simulink model "Simu_CA_CC_CC"  (R2024b)
settings: Solver=VariableStepAuto  StartTime=0.0  StopTime=10/60  RelTol=1e-3
libraries: spsDiodeLib x10, spsCurrentMeasurementLib x6, spsVoltageMeasurementLib x5, spsSeriesRLCBranchLib x2, spsACVoltageSourceLib x1, spsMeanLib x1, spsThreePhaseSourceLib x1, sps_lib x1
settings Model: Creator=usuario  LastModifiedBy=PC
settings OptimizationCC: ReuseModelBlockBuffer=off
settings RTWCC: GPUComputeCapability=3.5

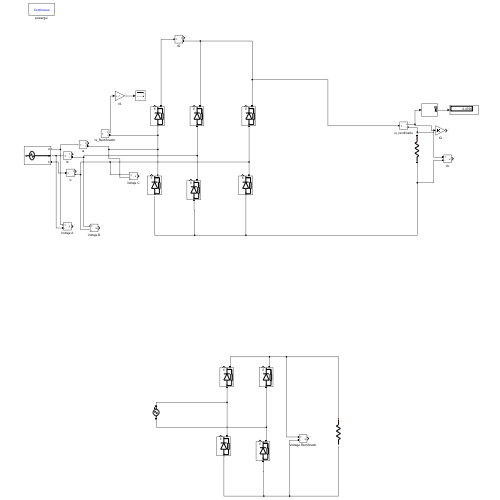
[thumbnail: Simulink's stored preview of the top-level diagram]
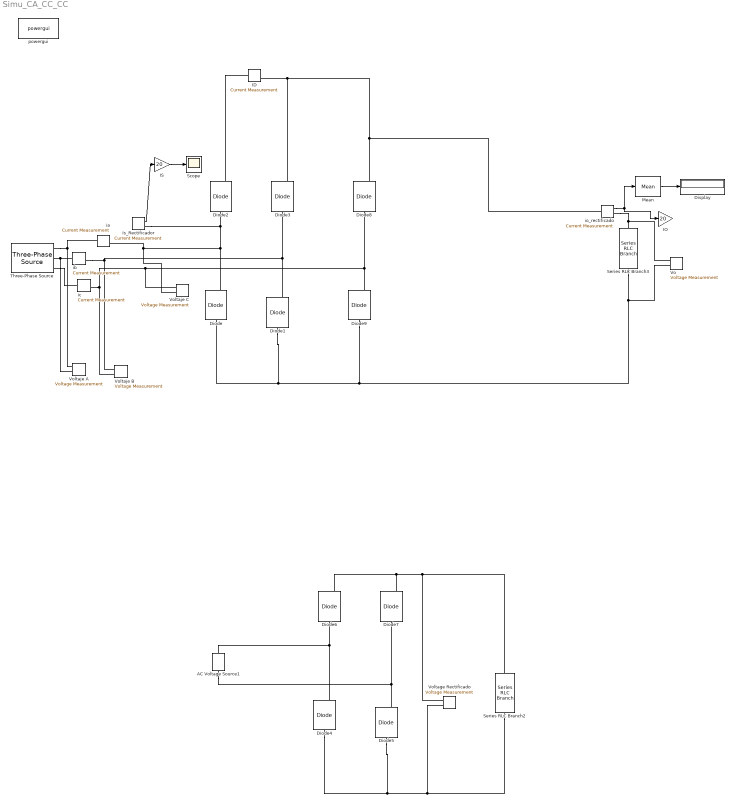
== system Simu_CA_CC_CC ==
  AC Voltage Source1 : spsACVoltageSourceLib/AC Voltage Source  Amplitude=105.56  Phase=0  Frequency=60  SampleTime=0  Measurements=None  BusType=swing  Pref=10e3  Qref=0  Qmin=-inf  Qmax=+inf
  Diode{,1..9} (10 alike) : spsDiodeLib/Diode  Ron=0.001  Lon=0  Vf=0.2  IC=0  UseSnubber=0  Rs=500  Cs=250e-9  Measurements=on
  Display : Display
  ID : spsCurrentMeasurementLib/Current Measurement  PhasorSimulation=off  OutputType=Complex  PSBequivalent=0
  IO : Gain  Gain=20
  IS : Gain  Gain=20
  Is_Rectificador : spsCurrentMeasurementLib/Current Measurement  PhasorSimulation=off  OutputType=Complex  PSBequivalent=0
  Mean : spsMeanLib/Mean  Freq=60  Vinit=0  Ts=0
  Scope : Scope
  Series RLC Branch2 : spsSeriesRLCBranchLib/Series RLC Branch  LConnTagsString=__new0  RConnTagsString=__new0  BranchType=R  Resistance=171  Inductance=1e-3  SetiL0=off  InitialCurrent=0  Capacitance=1e-6  Setx0=off  InitialVoltage=0  Measurements=Branch voltage and current
  Series RLC Branch3 : spsSeriesRLCBranchLib/Series RLC Branch  LConnTagsString=__new0  RConnTagsString=__new0  BranchType=R  Resistance=171  Inductance=1e-3  SetiL0=off  InitialCurrent=0  Capacitance=1e-6  Setx0=off  InitialVoltage=0  Measurements=Branch voltage and current
  Three-Phase Source : spsThreePhaseSourceLib/Three-Phase Source  InternalConnection=Yn  VoltagePhases=off  Voltage=60  PhaseAngle=0  Voltage_phases=[25e3 25e3 25e3]/sqrt(3)  PhaseAngles_phases=[0 -120 +120]  Frequency=60  NonIdealSource=on  SpecifyImpedance=off  Resistance=0  Inductance=0  ShortCircuitLevel=100e6  BaseVoltage=25e3  XRratio=7  BusType=swing  Pref=10e3  Qref=0  Prefabc=[10e3, 10e3, 10e3]  Qrefabc=[0, 0, 0]  Qmin=-inf  Qmax=inf
  Vo : spsVoltageMeasurementLib/Voltage Measurement  PhasorSimulation=off  OutputType=Complex  PSBequivalent=0
  Voltage Rectificado : spsVoltageMeasurementLib/Voltage Measurement  PhasorSimulation=off  OutputType=Complex  PSBequivalent=0
  Voltaje A : spsVoltageMeasurementLib/Voltage Measurement  PhasorSimulation=off  OutputType=Complex  PSBequivalent=0
  Voltaje B : spsVoltageMeasurementLib/Voltage Measurement  PhasorSimulation=off  OutputType=Complex  PSBequivalent=0
  Voltaje C : spsVoltageMeasurementLib/Voltage Measurement  PhasorSimulation=off  OutputType=Complex  PSBequivalent=0
  ia : spsCurrentMeasurementLib/Current Measurement  PhasorSimulation=off  OutputType=Complex  PSBequivalent=0
  ib : spsCurrentMeasurementLib/Current Measurement  PhasorSimulation=off  OutputType=Complex  PSBequivalent=0
  ic : spsCurrentMeasurementLib/Current Measurement  PhasorSimulation=off  OutputType=Complex  PSBequivalent=0
  io_rectificado : spsCurrentMeasurementLib/Current Measurement  PhasorSimulation=off  OutputType=Complex  PSBequivalent=0
  powergui : sps_lib/powergui  Priority=1  SimulationMode=Continuous  SampleTime=50e-6  frequency=60  Iterations=50  frequencyindice=60  Pbase=100e6  ErrMax=1e-4  UnitsV=kV  UnitsW=MW  buscounter=0  FunctionMessages=off  echomessages=off  EnableUseOfTLC=off  CurrentSourceSwitches=off  DisableSnubberDevices=off  DisableRonSwitches=off  DisableVfSwitches=off  DisplayEquations=off  AutomaticDiscreteSolvers=off  SolverType=Tustin/Backward Euler (TBE)  Interpol=off  ExternalGateDelay=off  methode=off  Ts=100  x0status=blocks  SPID=on  SwTol=0  HookPort=off  NonlinearTolerance=1e-4  nMaxIteration=100  ContinueOnMaxIteration=off  RestoreLinks=warning  ResistiveCurrentMeasurement=off  Frange=[0:2:500]  Ylog=off  Xlog=on  ShowGrid=off  save=off  variable=ZData  structure=0  ZoomFFT=off  StartTime=0.0  cycles=1  DisplayStyle=1  fundamental=60  FreqAxis=off  MaxFrequency=1000  frequencyindicesteady=1  RmsSteady=1  display=off
  wires:
  Mean/1 -> Display/1
  io_rectificado/1 -> IO/1, Mean/1
  Is_Rectificador/1 -> IS/1
  IS/1 -> Scope/1
  connections:
  Diode1/LConn1 -- Vo/LConn2 -- Series RLC Branch3/RConn1 -- Diode9/LConn1 -- Diode/LConn1
  Diode3/RConn1 -- io_rectificado/LConn1 -- Diode8/RConn1 -- ID/RConn1
  Diode/RConn1 -- ia/RConn1 -- Voltaje C/LConn2 -- Is_Rectificador/RConn1 -- Diode2/LConn1
  Diode1/RConn1 -- ib/RConn1 -- Voltaje B/LConn1 -- Diode3/LConn1
  Diode2/RConn1 -- ID/LConn1
  io_rectificado/RConn1 -- Vo/LConn1 -- Series RLC Branch3/LConn1
  AC Voltage Source1/LConn1 -- Diode5/RConn1 -- Diode7/LConn1
  Diode5/LConn1 -- Series RLC Branch2/RConn1 -- Voltage Rectificado/LConn2 -- Diode4/LConn1
  Diode7/RConn1 -- Diode6/RConn1 -- Series RLC Branch2/LConn1 -- Voltage Rectificado/LConn1
  Diode4/RConn1 -- AC Voltage Source1/RConn1 -- Diode6/LConn1
  Diode9/RConn1 -- Voltaje B/LConn2 -- ic/RConn1 -- Voltaje C/LConn1 -- Diode8/LConn1
  Three-Phase Source/RConn1 -- ia/LConn1 -- Voltaje A/LConn1
  Three-Phase Source/RConn2 -- ib/LConn1 -- Voltaje A/LConn2
  Three-Phase Source/RConn3 -- ic/LConn1
